simulink model "solargrid"  (R2021a)
settings: Solver=ode4  StartTime=0.0  StopTime=2.5  RelTol=1e-3
PreLoadFcn:
  | Ts_Power=1e-6;
  | Ts_Control=100e-6;
InitFcn:
  | Ts_Power=1e-6;
  | Ts_Control=100e-6;
undefined symbols (not defined in the file): D1, Delta, sigbuilder_block
libraries: spsSeriesRLCBranchLib x5, spsVoltageMeasurementLib x3, spsThreePhaseTransformerTwoWindingsLib x2, spsDistributedParametersLineLib x2, spsThreePhaseParallelRLCLoadLib x2, pid_lib x2, spsabctodq0Lib x2, spsThreePhaseSeriesRLCLoadLib x1, spsThreeLevelBridgeLib x1, spsThreePhaseSourceLib x1, spsGroundLib x1, spsGroundingTransformerLib x1
(part 1 of 2)
settings Model: SimulationMode=accelerator  Creator=The MathWorks, Inc.  LastModifiedBy=aks
settings SolverCC: AlgebraicLoopSolver=TrustRegion
settings DataIOCC: LimitDataPoints=on  SaveFormat=Array  SignalLogging=off  DSMLogging=off  ReturnWorkspaceOutputs=off
settings OptimizationCC: ExpressionDepthLimit=2147483647  EfficientMapNaN2IntZero=off  LifeSpan=inf
settings DebuggingCC: UnderspecifiedInitializationDetection=Classic  MergeDetectMultiDrivingBlocksExec=none  SolverPrmCheckMsg=warning  FcnCallInpInsideContextMsg=warning  StateNameClashWarn=warning  SFUnexpectedBacktrackingDiag=warning  SFNoUnconditionalDefaultTransitionDiag=warning  SFExecutionAtInitializationDiag=none  SFMachineParentedDataDiag=warning  ArithmeticOperatorsInVariantConditions=warning
settings HardwareCC: ProdBitPerPointer=32  ProdBitPerSizeT=32  ProdBitPerPtrDiffT=32  ProdLargestAtomicFloat=None  ProdIntDivRoundTo=Undefined  ProdEndianess=Unspecified  ProdWordSize=32  ProdHWDeviceType=32-bit Generic  TargetBitPerLong=64  TargetBitPerPointer=64  TargetBitPerSizeT=64  TargetBitPerPtrDiffT=64  TargetLongLongMode=on  TargetIntDivRoundTo=Zero  TargetEndianess=LittleEndian  TargetWordSize=64  TargetHWDeviceType=MATLAB Host  ProdEqTarget=off
settings ModelReferenceCC: PropagateSignalLabelsOutOfModel=off
settings SFSimCC: SimUseLocalCustomCode=off  CustomCodeUndefinedFunction=UseInterfaceOnly
settings CodeAppCC: MaxIdLength=128
settings GRTTargetCC: TargetLangStandard=C89/C90 (ANSI)  CombineOutputUpdateFcns=off  GRTInterface=on
settings ConfigComp: CovMetricSettings=dw  CovSaveCumulativeToWorkspaceVar=on  CovSaveSingleToWorkspaceVar=on  CovExternalEMLEnable=off  CovSFcnEnable=off
settings SimscapeCC: SimscapeNormalizeSystem=off

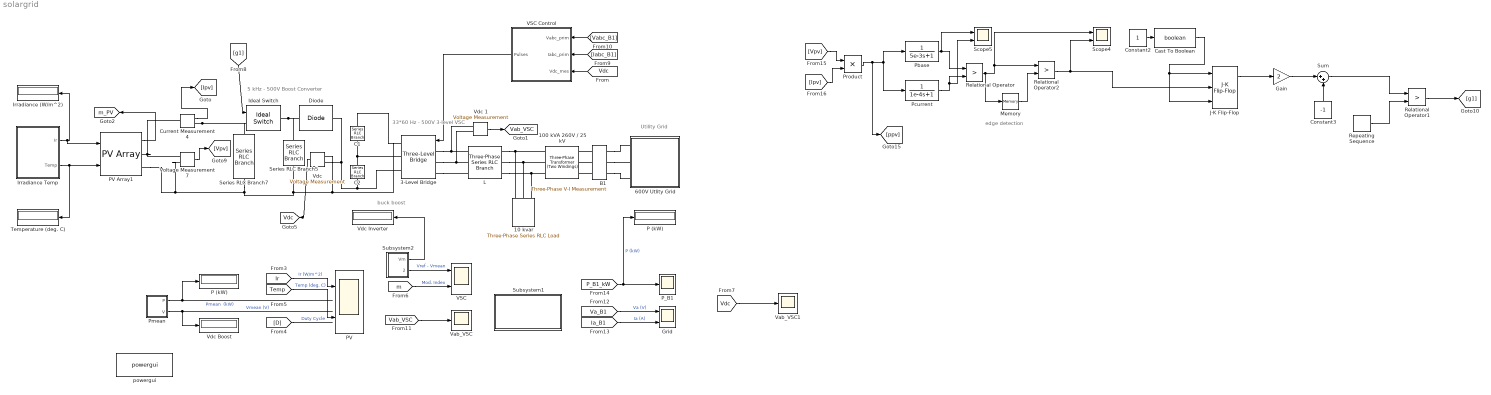
== system solargrid ==
  note: 5 kHz - 500V
      | Boost Converter
  note: 33*60 Hz - 500V
      | 3-level VSC
  note: Utility Grid
  note: buck boost
  note: edge detection
  10 kvar : spsThreePhaseSeriesRLCLoadLib/Three-Phase Series RLC Load  LConnTagsString=A|B|C  Configuration=Y (grounded)  NominalVoltage=240  Vabc=[1e3 1e3 1e3]  Vabcp=[1e3 1e3 1e3]  NominalFrequency=60  UnbalancedPower=off  ActivePower=10e3/100  InductivePower=0  CapacitivePower=10e3  Pabc=[10e3 9e3 11e3]  QLabc=[100 90 110]  QCabc=[100 90 110]  Pabcp=[10e3 9e3 11e3]  QLabcp=[100 90 110]  QCabcp=[100 90 110]  Measurements=None  LoadType=constant Z
  100 kVA 260V / 25 kV : spsThreePhaseTransformerTwoWindingsLib/Three-Phase Transformer (Two Windings)  Winding1Connection=Yg  Winding2Connection=Delta (D1)  CoreType=Three single-phase transformers  SetSaturation=off  Hysteresis=off  DataFile='hysteresis'  SetInitialFlux=off  Measurements=None  UNITS=pu  NominalPower=[100e3 , 60 ]  Winding1=[ 25e3 , 0.001 , 0.03 ]  Winding2=[ 260 , 0.001 , 0.03 ]  Rm=500  Lm=500  L0=0.5  Saturation=[ 0,0 ; 0.0024,1.2 ; 1.0,1.52 ]  InitialFluxes=[ 0.8 , -0.8 , 0.7 ]  BreakLoop=off  DiscreteSolver=Trapezoidal iterative  DataType=off  TransfoNumber=0
  3-Level Bridge : spsThreeLevelBridgeLib/Three-Level Bridge  Arms=3  SnubberResistance=1e6  SbubberCapacitance=inf  Device=IGBT / Diodes  Ron=0.2e-3  ForwardVoltages="[  0  0 ]"  Measurements=None
      settings: AttributesFormatString=\n  SourceProductBaseCode=PS
  600V Utlity Grid : Subsystem
  B1 : spsThreePhaseVIMeasurementLib/Three-Phase V-I Measurement  VoltageMeasurement=phase-to-ground  SetLabelV=on  LabelV=Vabc_B1  Vpu=off  VpuLL=off  CurrentMeasurement=yes  SetLabelI=on  LabelI=Iabc_B1  Ipu=off  Pbase=100e6  Vbase=500e3  OutputType=Magnitude  PhasorSimulation=off  PSBequivalent=0
  C1 : spsSeriesRLCBranchLib/Series RLC Branch  LConnTagsString=__new0  RConnTagsString=__new0  BranchType=C  Resistance=1.0  Inductance=1.0  SetiL0=off  InitialCurrent=0  Capacitance=12000e-06  Setx0=off  InitialVoltage=0  Measurements=None
  C2 : spsSeriesRLCBranchLib/Series RLC Branch  LConnTagsString=__new0  RConnTagsString=__new0  BranchType=C  Resistance=1.0  Inductance=1.0  SetiL0=off  InitialCurrent=0  Capacitance=12000e-06  Setx0=off  InitialVoltage=0  Measurements=None
  Cast To Boolean : DataTypeConversion  OutDataTypeStr=boolean
  Constant2 : Constant
  Constant3 : Constant  Value=-1
  Current Measurement4 : spsCurrentMeasurementLib/Current Measurement  PhasorSimulation=off  OutputType=Complex  PSBequivalent=0
  Diode : spsDiodeLib/Diode  Ron=1e-5  Lon=0  Vf=0.8  IC=0  UseSnubber=0  Rs=500  Cs=250e-9  Measurements=off
  Gain : Gain  Gain=2
  Grid : Scope  NumInputPorts=2
  Ideal Switch : spsIdealSwitchLib/Ideal Switch  Ron=0.001  Lon=0  IC=0  Rs=1e5  Cs=inf  Measurements=off
  Irradiance (W/m^2) : Display
      settings: Format=bank  Decimation=1000
  Irradiance Temp : Subsystem  Tag=STV Subsys  LoadFcn=sigbuilder_block('load');  StartFcn=sigbuilder_block('start');  StopFcn=sigbuilder_block('stop');  ClipboardFcn=sigbuilder_block('clipboard');  mask(Sigbuilder block){tuvar=[0:10]}
      mask help: Sigbuilder GUI
      mask init:
      | if ~strcmp(get_param(bdroot(gcbh),'SimulationStatus'),'stopped') tuvar = sigbuilder_block('maskInit'); end
      settings: CopyFcn=sigbuilder_block('copy');  DeleteFcn=sigbuilder_block('delete');  ModelCloseFcn=sigbuilder_block('modelClose');  PreSaveFcn=sigbuilder_block('preSave');  PauseFcn=sigbuilder_block('pause')  ContinueFcn=sigbuilder_block('continue')  NameChangeFcn=sigbuilder_block('namechange');  OpenFcn=sigbuilder_block('open',[54 0 1386 674.25 ]);  CloseFcn=sigbuilder_block('close');
      mask Display: plot(0, 0, 100, 100,[2, 2, 32, 32, 2], [68, 8, 8, 68, 68],[32, 2], [38, 38], [32, 19, 2],[53, 60, 44], [32, 17, 17, 2],[16, 16, 31, 31]);txt = getActiveGroup(gcbh);text(2, 100, txt,'verticalAlignment', 'top');
  J-K Flip-Flop : simulink_extras/Flip Flops/J-K Flip-Flop  initial_condition=1
  L : spsThreePhaseSeriesRLCBranchLib/Three-Phase Series RLC Branch  LConnTagsString=A|B|C  RConnTagsString=A|B|C  BranchType=RL  Resistance=500e-6*377/50/2  Inductance=500e-6/2  Capacitance=inf  Measurements=None
  Memory : Memory  InheritSampleTime=on
  P (kW) : Display
      settings: Format=bank  Decimation=2000
  "P (kW) " : Display
      settings: Format=bank  Decimation=2000
  PV : Scope  NumInputPorts=2
  PV Array1 : spsPVArrayLib/PV Array  Npar=40  Nser=10  PlotType=array @ 1000 W/m2 & specified temperatures  S_vec="[ 1000  500  100 ]"  Temp_C_vec=[ 45 25]  ModuleName=User-defined  PlotWhenSelected=off  Pm=213.15  Ncell=60  Voc=36.3  Isc=7.84  Vm=29  Im=7.35  beta_Voc_pc=-0.36099  alpha_Isc_pc=0.102  beta_Voc=-0.13104  alpha_Isc=0.0079968  IL=7.8654  I0=2.9273e-10  nI=0.98119  Rsh=313.0553  Rs=0.39381  RobustModel=off  RobustCellTemperature=313.3991  BAL=on  Tc=1e-6  Tfilter=5e-5
  P_B1 : Scope
  Pbase : TransferFcn  Denominator=[5e-3 1]
  Pcurrent : TransferFcn  Denominator=[1e-4 1]
  Pmean : Subsystem
  Product : Product
  Relational Operator : RelationalOperator  Operator=>  OutDataTypeStr=boolean  RndMeth=Simplest
  Relational Operator1 : RelationalOperator  Operator=>  OutDataTypeStr=boolean  RndMeth=Simplest
  Relational Operator2 : RelationalOperator  Operator=>  OutDataTypeStr=boolean  RndMeth=Simplest
  Repeating Sequence : simulink/Sources/Repeating Sequence  rep_seq_t=[0 1/40e3 1/20e3 3/40e3 1/10e3]  rep_seq_y=[0 1 0 -1 0]
  Scope4 : Scope  NumInputPorts=2
  Scope5 : Scope  NumInputPorts=2
  Series RLC Branch5 : spsSeriesRLCBranchLib/Series RLC Branch  LConnTagsString=__new0  RConnTagsString=__new0  BranchType=L  Resistance=1  Inductance=10e-3  SetiL0=off  InitialCurrent=0  Capacitance=1e-6  Setx0=off  InitialVoltage=0  Measurements=None
  Series RLC Branch7 : spsSeriesRLCBranchLib/Series RLC Branch  LConnTagsString=__new0  RConnTagsString=__new0  BranchType=C  Resistance=1  Inductance=1e-3  SetiL0=off  InitialCurrent=0  Capacitance=100e-6  Setx0=off  InitialVoltage=0  Measurements=None
  Subsystem1 : Subsystem
      mask Display: disp('Open this block\nto display additional \nscopes & measurements')
  Subsystem2 : Subsystem
  Sum : Sum  Inputs=|++
  Temperature (deg. C) : Display
      settings: Format=bank  Decimation=1000
  VSC : Scope  NumInputPorts=2
  VSC Control : Subsystem  mask(VSC Main Controller){nom=[ 100e3  60 ], Vnom=[ 25e3 260 ], Vnom_dc=500, RLxfo=[0.002  0.06 ], RLchoke=[2e-3  250e-6  ], K_VDCreg=[7  800], K_Ireg=[0.3 20], Ts=Ts_Control}
      mask prompts: nom "Nominal power and frequency [ Pnom(VA)  Fnom(Hz) ]:"; Vnom "Nominal primary and secondary voltages (Vrms LL) [ Vnom_prim   Vnom_sec ]:"; Vnom_dc "Nominal DC bus voltage (V):"; RLxfo "Total transformer leakage impedance (pu/Pnom) [ Rxfo  Lxf ]"; RLchoke "Choke impedance [ R(ohm) L(H) ]"; K_VDCreg "VDC regultator gains [ Kp  Ki ]:"; K_Ireg "Current regulator gains [ Kp  Ki ]:"; Ts "Sample time"
      mask init:
      | Pnom=nom(1);
      | Fnom=nom(2);
      | Vnom_prim=Vnom(1);
      | Vnom_sec=Vnom(2);
      | Zbase=Vnom_sec^2/Pnom;
      | Rtot_pu=RLxfo(1) + RLchoke(1)/Zbase;
      | Ltot_pu=RLxfo(2) + RLchoke(2)/(Zbase/(2*pi*Fnom));
      | Kp_VDCreg=K_VDCreg(1);
      | Ki_VDCreg=K_VDCreg(2);
      | Kp_Ireg=K_Ireg(1);
      | Ki_Ireg=K_Ireg(2);
      | Vdc_ref=Vnom_dc;
      | % Used to determine initial value of Boost Control (MPPT)
      | assignin('base','Vdc_ref_Inv',Vdc_ref);
  Vab_VSC : Scope
  Vab_VSC1 : Scope
  "Vdc " : spsVoltageMeasurementLib/Voltage Measurement  Tag=PoWeRsYsTeMmEaSuReMeNt  PhasorSimulation=off  OutputType=Magnitude  PSBequivalent=0
  Vdc 1 : spsVoltageMeasurementLib/Voltage Measurement  Tag=PoWeRsYsTeMmEaSuReMeNt  PhasorSimulation=off  OutputType=Magnitude  PSBequivalent=0
  Vdc Boost : Display
      settings: Format=bank  Decimation=2000
  Vdc Inverter : Display
      settings: Format=bank  Decimation=2000
  Voltage Measurement7 : spsVoltageMeasurementLib/Voltage Measurement  PhasorSimulation=off  OutputType=Complex  PSBequivalent=0
  powergui : spspowerguiLib/powergui  Priority=1  SimulationMode=Discrete  SampleTime=1e-06  frequency=60  Iterations=50  frequencyindice=0  Pbase=100e6  ErrMax=1e-4  UnitsV=kV  UnitsW=MW  buscounter=0  FunctionMessages=off  echomessages=off  EnableUseOfTLC=off  CurrentSourceSwitches=off  DisableSnubberDevices=off  DisableRonSwitches=off  DisableVfSwitches=off  DisplayEquations=off  AutomaticDiscreteSolvers=off  SolverType=Tustin/Backward Euler (TBE)  Interpol=off  ExternalGateDelay=off  methode=off  Ts=0  x0status=blocks  SPID=off  SwTol=0  HookPort=off  NonlinearTolerance=1e-8  nMaxIteration=10  ContinueOnMaxIteration=off  RestoreLinks=warning  ResistiveCurrentMeasurement=off  Frange=[0:2:500]  Ylog=off  Xlog=on  ShowGrid=off  save=off  variable=ZData  structure=0  ZoomFFT=on  StartTime=0.0  cycles=1  DisplayStyle=1  fundamental=60  FreqAxis=off  MaxFrequency=1000  frequencyindicesteady=1  RmsSteady=1  display=off
  tag scope: Vab_VSC=global, Vdc=global, m_PV=global
  wires:
  "Vdc "/1 -> [Vdc]
  [Vabc_B1] -> VSC Control/1(Vabc_prim)
  [Iabc_B1] -> VSC Control/2(Iabc_prim)
  [Vdc] -> VSC Control/3(Vdc_mes)
  VSC Control/1(Pulses) -> 3-Level Bridge/1
  Pmean/1(P) -> "P (kW) "/1  "Pmean  (kW)"
  [m] -> VSC/2  "Mod. Index"
  Vdc 1/1 -> [Vab_VSC]
  [Vab_VSC] -> Vab_VSC/1
  [Ia_B1] -> Grid/2  "Ia (A)"
  [Va_B1] -> Grid/1  "Va (V)"
  [P_B1_kW] -> P_B1/1, P (kW)/1  "P (kW)"
  Pmean/2(V) -> Vdc Boost/1  "Vmean (V)"
  Subsystem2/2(VrVm) -> VSC/1  "Vref - Vmean"
  Subsystem2/1(Vm) -> Vdc Inverter/1
  Irradiance Temp/1(Ir) -> PV Array1/1, Irradiance (W/m^2)/1
  Irradiance Temp/2(Temp) -> PV Array1/2, Temperature (deg. C)/1
  [D] -> ?  "Duty Cycle"
  [Temp] -> PV/2  "Temp (deg. C)"
  [Ir] -> PV/1  "Ir (W/m^2)"
  PV Array1/1 -> [m_PV]
  [Vdc] -> Vab_VSC1/1
  Voltage Measurement7/1 -> [Vpv]
  [g1] -> Ideal Switch/1
  Current Measurement4/1 -> [Ipv]
  Relational Operator1/1 -> [g1]
  Product/1 -> [ppv], Pcurrent/1, Pbase/1
  [Vpv] -> Product/1
  Constant2/1 -> Cast To Boolean/1
  Relational Operator2/1 -> Scope4/2, J-K Flip-Flop/2
  Constant3/1 -> Sum/2
  Relational Operator/1 -> Scope4/1, Relational Operator2/1, Memory/1
  Pbase/1 -> Scope5/1, Relational Operator/1
  Memory/1 -> Relational Operator2/2
  Cast To Boolean/1 -> J-K Flip-Flop/3, J-K Flip-Flop/1
  [Ipv] -> Product/2
  Sum/1 -> Relational Operator1/1
  Gain/1 -> Sum/1
  Pcurrent/1 -> Scope5/2, Relational Operator/2
  Repeating Sequence/1 -> Relational Operator1/2
  J-K Flip-Flop/1 -> Gain/1
  connections:
  3-Level Bridge/LConn1 -- L/LConn1 -- Vdc 1/LConn1
  3-Level Bridge/LConn2 -- L/LConn2 -- Vdc 1/LConn2
  3-Level Bridge/LConn3 -- L/LConn3
  L/RConn1 -- 100 kVA 260V / 25 kV/RConn1 -- 10 kvar/LConn1
  L/RConn2 -- 100 kVA 260V / 25 kV/RConn2 -- 10 kvar/LConn2
  L/RConn3 -- 100 kVA 260V / 25 kV/RConn3 -- 10 kvar/LConn3
  B1/LConn1 -- 100 kVA 260V / 25 kV/LConn1
  B1/LConn2 -- 100 kVA 260V / 25 kV/LConn2
  B1/LConn3 -- 100 kVA 260V / 25 kV/LConn3
  C2/LConn1 -- C1/RConn1 -- 3-Level Bridge/RConn2
  B1/RConn2 -- 600V Utlity Grid/LConn2
  B1/RConn1 -- 600V Utlity Grid/LConn1
  B1/RConn3 -- 600V Utlity Grid/LConn3
  Current Measurement4/RConn1 -- Series RLC Branch7/LConn1 -- Ideal Switch/LConn1
  Ideal Switch/RConn1 -- Series RLC Branch5/LConn1 -- Diode/RConn1
  Voltage Measurement7/LConn1 -- PV Array1/RConn1 -- Current Measurement4/LConn1
  Voltage Measurement7/LConn2 -- Series RLC Branch7/RConn1 -- "Vdc "/LConn1 -- 3-Level Bridge/RConn1 -- C1/LConn1 -- Series RLC Branch5/RConn1 -- PV Array1/RConn2
  Diode/LConn1 -- "Vdc "/LConn2 -- C2/RConn1 -- 3-Level Bridge/RConn3

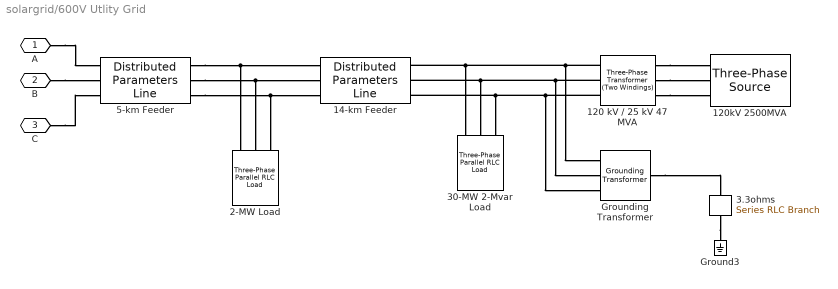
== system solargrid/600V Utlity Grid ==
  120 kV / 25 kV 47 MVA : spsThreePhaseTransformerTwoWindingsLib/Three-Phase Transformer (Two Windings)  Winding1Connection=Yg  Winding2Connection=Delta (D1)  CoreType=Three single-phase transformers  SetSaturation=off  Hysteresis=off  DataFile='basic_model'  SetInitialFlux=off  Measurements=None  UNITS=pu  NominalPower=[47e6 60 ]  Winding1="[ 120e3  0.08/30   0.08 ]"  Winding2="[ 25e3  0.08/30  0.08]"  Rm=500  Lm=500  L0=0.5  Saturation="[ 0,0  ;  0.005,1.2  ;  1.0,1.4 ]"  InitialFluxes=[ 0.8 , -0.8 , 0.7 ]  BreakLoop=off  DiscreteSolver=Trapezoidal iterative  DataType=off  TransfoNumber=0
  120kV 2500MVA : spsThreePhaseSourceLib/Three-Phase Source  InternalConnection=Yg  VoltagePhases=off  Voltage=120e3  PhaseAngle=0  Voltage_phases=[25e3 25e3 25e3]/sqrt(3)  PhaseAngles_phases=[0 -120 +120]  Frequency=60  NonIdealSource=on  SpecifyImpedance=on  Resistance=0.8929  Inductance=16.58e-3  ShortCircuitLevel=2500e6  BaseVoltage=120e3  XRratio=7  BusType=swing  Pref=0  Qref=0  Prefabc=[10e3, 10e3, 10e3]  Qrefabc=[0, 0, 0]  Qmin=-inf  Qmax=inf
  14-km Feeder : spsDistributedParametersLineLib/Distributed Parameters Line  Phases=3  Length=14  Frequency=60  Resistance=[0.1153 0.413]  Inductance=[1.05e-3 3.32e-3]  Capacitance=[11.33e-009 5.01e-009]  x1=[-5.8e-05 -4.281464951191e-09 0 0;-5.7e-05 -4.28163095328358e-09 0 0;-5.6e-05 -4.28179634686092e-09 0 0;-5.5e-05 -4.28196113189951e-09 0 0;-5.4e-05 -4.28212530837592e-09 0 0;-5.3e-05 -4.28228887626683e-09 0 0;-5.2e-05 -4.28245183554898e-09 0 0;-5.1e-05 -4.28261418619923e-09 0 0;-5e-05 -4.28277592819449e-09 0 0;-4.9e-05 -4.28293706151177e-09 -3790.73535189767 -24061.4134200266;-4.8e-05 -4.28309758612819e-09 -3781.66414358227 -24062.840783721;-4.7e-05 -4.28325750202091e-09 -3772.59239780806 -24064.2647275491;-4.6e-05 -4.28341680916722e-09 -3763.52011586434 -24065.6852513085;-4.5e-05 -4.28357550754448e-09 -3754.44729904048 -24067.1023547973;-4.4e-05 -4.28373359713012e-09 -3745.37394862592 -24068.5160378142;-4.3e-05 -4.28389107790169e-09 -3736.3000659102 -24069.9263001581;-4.2e-05 -4.2840479498368e-09 -3727.22565218291 -24071.3331416287;-4.1e-05 -4.28420421291315e-09 -3718.15070873374 -24072.7365620261;-4e-05 -4.28435986710853e-09 -3709.07523685243 -24074.1365611507;-3.9e-05 -4.28451491240084e-09 -3699.9992378288 -24075.5331388036;-3.8e-05 -4.28466934876802e-09 -3690.92271295277 -24076.9262947863;-3.7e-05 -4.28482317618813e-09 -3681.84566351431 -24078.3160289009;-3.6e-05 -4.2849763946393e-09 -3672.76809080347 -24079.7023409497;-3.5e-05 -4.28512900409978e-09 -3663.68999611037 -24081.0852307359;-3.4e-05 -4.28528100454785e-09 -3654.61138072522 -24082.4646980627;-3.3e-05 -4.28543239596192e-09 -3645.53224593829 -24083.8407427343;-3.2e-05 -4.28558317832048e-09 -3636.45259303993 -24085.213364555;-3.1e-05 -4.28573335160209e-09 -3627.37242332055 -24086.5825633297;-3e-05 -4.28588291578542e-09 -3618.29173807065 -24087.9483388638;-2.9e-05 -4.2860318708492e-09 -3609.2105385808 -24089.3106909633;-2.8e-05 -4.28618021677226e-09 -3600.12882614165 -24090.6696194346;-2.7e-05 -4.28632795353353e-09 -3591.0466020439 -24092.0251240844;-2.6e-05 -4.286475081112e-09 -3581.96386757834 -24093.3772047201;-2.5e-05 -4.28662159948677e-09 -3572.88062403583 -24094.7258611496;-2.4e-05 -4.28676750863701e-09 -3563.7968727073 -24096.0710931813;-2.3e-05 -4.28691280854198e-09 -3554.71261488376 -24097.4129006238;-2.2e-05 -4.28705749918104e-09 -3545.62785185628 -24098.7512832866;-2.1e-05 -4.28720158053362e-09 -3536.54258491601 -24100.0862409793;-2e-05 -4.28734505257924e-09 -3527.45681535417 -24101.4177735123;-1.9e-05 -4.28748791529752e-09 -3518.37054446204 -24102.7458806964;-1.8e-05 -4.28763016866814e-09 -3509.283773531 -24104.0705623427;-1.7e-05 -4.2877718126709e-09 -3500.19650385247 -24105.3918182631;-1.6e-05 -4.28791284728566e-09 -3491.10873671795 -24106.7096482696;-1.5e-05 -4.28805327249237e-09 -3482.02047341903 -24108.0240521751;-1.4e-05 -4.28819308827108e-09 -3472.93171524734 -24109.3350297928;-1.3e-05 -4.28833229460192e-09 -3463.8424634946 -24110.6425809363;-1.2e-05 -4.28847089146511e-09 -3454.7527194526 -24111.9467054197;-1.1e-05 -4.28860887884094e-09 -3445.66248441319 -24113.2474030578;-1e-05 -4.28874625670981e-09 -3436.5717596683 -24114.5446736656;-9e-06 -4.28888302505218e-09 -3427.48054650992 -24115.8385170589;-8e-06 -4.28901918384863e-09 -3418.38884623011 -24117.1289330537;-7e-06 -4.2891547330798e-09 -3409.29666012101 -24118.4159214666;-6e-06 -4.28928967272643e-09 -3400.20398947483 -24119.6994821147;-5e-06 -4.28942400276934e-09 -3391.11083558383 -24120.9796148156;-4e-06 -4.28955772318944e-09 -3382.01719974035 -24122.2563193874;-3e-06 -4.28969083396771e-09 -3372.9230832368 -24123.5295956486;-2e-06 -4.28982333508526e-09 -3363.82848736566 -24124.7994434182;-1e-06 -4.28995522652324e-09 -3354.73341341947 -24126.0658625158]  x2=[-5.8e-05 -4.62050791098548e-09 0 0;-5.7e-05 -4.62061598144239e-09 0 0;-5.6e-05 -4.62072339520672e-09 0 0;-5.5e-05 -4.6208301522632e-09 0 0;-5.4e-05 -4.62093625259667e-09 0 0;-5.3e-05 -4.62104169619204e-09 0 0;-5.2e-05 -4.62114648303433e-09 0 0;-5.1e-05 -4.62125061310864e-09 0 0;-5e-05 -4.62135408640018e-09 0 0;-4.9e-05 -4.62145690289425e-09 -3379.39242591114 -24244.0512732168;-4.8e-05 -4.62155906257621e-09 -3370.25239397934 -24245.3235513067;-4.7e-05 -4.62166056543157e-09 -3361.11188305951 -24246.5923835954;-4.6e-05 -4.62176141144589e-09 -3351.97089445072 -24247.8577699026;-4.5e-05 -4.62186160060484e-09 -3342.82942945211 -24249.1197100484;-4.4e-05 -4.62196113289418e-09 -3333.68748936289 -24250.3782038535;-4.3e-05 -4.62206000829977e-09 -3324.54507548233 -24251.6332511391;-4.2e-05 -4.62215822680755e-09 -3315.40218910977 -24252.8848517267;-4.1e-05 -4.62225578840356e-09 -3306.25883154462 -24254.1330054385;-4e-05 -4.62235269307394e-09 -3297.11500408636 -24255.3777120971;-3.9e-05 -4.62244894080492e-09 -3287.97070803452 -24256.6189715256;-3.8e-05 -4.62254453158282e-09 -3278.82594468872 -24257.8567835476;-3.7e-05 -4.62263946539405e-09 -3269.68071534863 -24259.0911479871;-3.6e-05 -4.62273374222511e-09 -3260.53502131399 -24260.3220646688;-3.5e-05 -4.62282736206262e-09 -3251.38886388461 -24261.5495334176;-3.4e-05 -4.62292032489326e-09 -3242.24224436036 -24262.7735540592;-3.3e-05 -4.62301263070382e-09 -3233.09516404117 -24263.9941264196;-3.2e-05 -4.62310427948119e-09 -3223.94762422707 -24265.2112503252;-3.1e-05 -4.62319527121234e-09 -3214.7996262181 -24266.4249256032;-3e-05 -4.62328560588433e-09 -3205.65117131441 -24267.6351520811;-2.9e-05 -4.62337528348434e-09 -3196.5022608162 -24268.8419295867;-2.8e-05 -4.6234643039996e-09 -3187.35289602373 -24270.0452579487;-2.7e-05 -4.62355266741748e-09 -3178.20307823734 -24271.245136996;-2.6e-05 -4.62364037372541e-09 -3169.0528087574 -24272.4415665581;-2.5e-05 -4.62372742291093e-09 -3159.90208888438 -24273.6345464649;-2.4e-05 -4.62381381496166e-09 -3150.75091991881 -24274.8240765469;-2.3e-05 -4.62389954986533e-09 -3141.59930316127 -24276.010156635;-2.2e-05 -4.62398462760976e-09 -3132.4472399124 -24277.1927865607;-2.1e-05 -4.62406904818285e-09 -3123.29473147291 -24278.3719661559;-2e-05 -4.6241528115726e-09 -3114.1417791436 -24279.547695253;-1.9e-05 -4.62423591776711e-09 -3104.98838422528 -24280.7199736848;-1.8e-05 -4.62431836675457e-09 -3095.83454801887 -24281.8888012849;-1.7e-05 -4.62440015852325e-09 -3086.68027182533 -24283.054177887;-1.6e-05 -4.62448129306155e-09 -3077.52555694568 -24284.2161033256;-1.5e-05 -4.62456177035791e-09 -3068.37040468102 -24285.3745774355;-1.4e-05 -4.62464159040092e-09 -3059.21481633249 -24286.529600052;-1.3e-05 -4.62472075317922e-09 -3050.05879320131 -24287.6811710111;-1.2e-05 -4.62479925868155e-09 -3040.90233658876 -24288.829290149;-1.1e-05 -4.62487710689678e-09 -3031.74544779616 -24289.9739573026;-1e-05 -4.62495429781382e-09 -3022.58812812493 -24291.1151723092;-9e-06 -4.62503083142172e-09 -3013.43037887651 -24292.2529350066;-8e-06 -4.62510670770958e-09 -3004.27220135243 -24293.3872452331;-7e-06 -4.62518192666664e-09 -2995.11359685428 -24294.5181028274;-6e-06 -4.62525648828219e-09 -2985.95456668368 -24295.645507629;-5e-06 -4.62533039254565e-09 -2976.79511214235 -24296.7694594775;-4e-06 -4.62540363944651e-09 -2967.63523453204 -24297.8899582131;-3e-06 -4.62547622897435e-09 -2958.47493515459 -24299.0070036768;-2e-06 -4.62554816111886e-09 -2949.31421531186 -24300.1205957096;-1e-06 -4.62561943586983e-09 -2940.15307630582 -24301.2307341534]  x3=[-5.8e-05 -1.8600557383193e-11 0 0;-5.7e-05 -1.86061131377125e-11 0 0;-5.6e-05 -1.86116662478883e-11 0 0;-5.5e-05 -1.86172167129313e-11 0 0;-5.4e-05 -1.86227645320527e-11 0 0;-5.3e-05 -1.86283097044638e-11 0 0;-5.2e-05 -1.86338522293767e-11 0 0;-5.1e-05 -1.86393921060037e-11 0 0;-5e-05 -1.86449293335573e-11 0 0;-4.9e-05 -1.86504639112507e-11 -23.5442847382522 -155.681477773836;-4.8e-05 -1.86559958382971e-11 -23.4855925321335 -155.690342696957;-4.7e-05 -1.86615251139106e-11 -23.4268969881884 -155.699185493008;-4.6e-05 -1.86670517373051e-11 -23.3681981147587 -155.708006160732;-4.5e-05 -1.86725757076953e-11 -23.3094959201869 -155.716804698877;-4.4e-05 -1.8678097024296e-11 -23.2507904128159 -155.72558110619;-4.3e-05 -1.86836156863226e-11 -23.1920816009891 -155.734335381426;-4.2e-05 -1.86891316929907e-11 -23.1333694930502 -155.743067523339;-4.1e-05 -1.86946450435164e-11 -23.0746540973437 -155.751777530689;-4e-05 -1.87001557371162e-11 -23.0159354222141 -155.760465402238;-3.9e-05 -1.87056637730067e-11 -22.9572134760069 -155.769131136751;-3.8e-05 -1.87111691504053e-11 -22.8984882670676 -155.777774732997;-3.7e-05 -1.87166718685294e-11 -22.8397598037425 -155.786396189746;-3.6e-05 -1.87221719265971e-11 -22.7810280943782 -155.794995505775;-3.5e-05 -1.87276693238266e-11 -22.7222931473217 -155.80357267986;-3.4e-05 -1.87331640594366e-11 -22.6635549709206 -155.812127710783;-3.3e-05 -1.87386561326462e-11 -22.6048135735229 -155.820660597328;-3.2e-05 -1.87441455426749e-11 -22.546068963477 -155.829171338281;-3.1e-05 -1.87496322887424e-11 -22.487321149132 -155.837659932435;-3e-05 -1.87551163700691e-11 -22.4285701388371 -155.846126378581;-2.9e-05 -1.87605977858755e-11 -22.3698159409422 -155.854570675517;-2.8e-05 -1.87660765353825e-11 -22.3110585637976 -155.862992822043;-2.7e-05 -1.87715526178115e-11 -22.2522980157539 -155.871392816961;-2.6e-05 -1.87770260323843e-11 -22.1935343051625 -155.879770659078;-2.5e-05 -1.87824967783229e-11 -22.1347674403749 -155.888126347204;-2.4e-05 -1.87879648548499e-11 -22.0759974297432 -155.89645988015;-2.3e-05 -1.8793430261188e-11 -22.0172242816199 -155.904771256733;-2.2e-05 -1.87988929965606e-11 -21.958448004358 -155.91306047577;-2.1e-05 -1.88043530601912e-11 -21.899668606311 -155.921327536085;-2e-05 -1.88098104513039e-11 -21.8408860958326 -155.929572436502;-1.9e-05 -1.8815265169123e-11 -21.7821004812773 -155.937795175848;-1.8e-05 -1.88207172128734e-11 -21.7233117709996 -155.945995752957;-1.7e-05 -1.88261665817801e-11 -21.664519973355 -155.954174166662;-1.6e-05 -1.88316132750686e-11 -21.6057250966988 -155.9623304158;-1.5e-05 -1.8837057291965e-11 -21.5469271493873 -155.970464499213;-1.4e-05 -1.88424986316954e-11 -21.4881261397769 -155.978576415745;-1.3e-05 -1.88479372934865e-11 -21.4293220762246 -155.986666164242;-1.2e-05 -1.88533732765654e-11 -21.3705149670877 -155.994733743556;-1.1e-05 -1.88588065801595e-11 -21.311704820724 -156.002779152538;-1e-05 -1.88642372034965e-11 -21.2528916454918 -156.010802390047;-9e-06 -1.88696651458048e-11 -21.1940754497497 -156.018803454941;-8e-06 -1.88750904063129e-11 -21.1352562418568 -156.026782346084;-7e-06 -1.88805129842496e-11 -21.0764340301726 -156.034739062342;-6e-06 -1.88859328788444e-11 -21.0176088230572 -156.042673602583;-5e-06 -1.88913500893269e-11 -20.9587806288708 -156.05058596568;-4e-06 -1.88967646149273e-11 -20.8999494559742 -156.058476150509;-3e-06 -1.8902176454876e-11 -20.8411153127287 -156.066344155948;-2e-06 -1.89075856084039e-11 -20.782278207496 -156.074189980879;-1e-06 -1.89129920747421e-11 -20.723438148638 -156.082013624187]  x4=[-5.8e-05 7.79859018799454e-12 0 0;-5.7e-05 7.80427695538787e-12 0 0;-5.6e-05 7.80996261361939e-12 0 0;-5.5e-05 7.81564716188105e-12 0 0;-5.4e-05 7.82133059936495e-12 0 0;-5.3e-05 7.82701292526334e-12 0 0;-5.2e-05 7.83269413876864e-12 0 0;-5.1e-05 7.83837423907342e-12 0 0;-5e-05 7.84405322537041e-12 0 0;-4.9e-05 7.8497310968525e-12 -1.3558136600917 -2.15298522697949;-4.8e-05 7.85540785271274e-12 -1.35500190745656 -2.15349620368187;-4.7e-05 7.86108349214434e-12 -1.35418996224543 -2.15400687432443;-4.6e-05 7.86675801434066e-12 -1.35337782457371 -2.15451723883456;-4.5e-05 7.87243141849522e-12 -1.35256549455682 -2.15502729713975;-4.4e-05 7.87810370380171e-12 -1.3517529723102 -2.1555370491675;-4.3e-05 7.88377486945396e-12 -1.35094025794934 -2.15604649484536;-4.2e-05 7.88944491464599e-12 -1.35012735158974 -2.15655563410093;-4.1e-05 7.89511383857194e-12 -1.34931425334694 -2.15706446686185;-4e-05 7.90078164042615e-12 -1.34850096333649 -2.1575729930558;-3.9e-05 7.90644831940308e-12 -1.34768748167397 -2.15808121261052;-3.8e-05 7.91211387469738e-12 -1.34687380847501 -2.15858912545376;-3.7e-05 7.91777830550384e-12 -1.34605994385525 -2.15909673151335;-3.6e-05 7.92344161101743e-12 -1.34524588793034 -2.15960403071714;-3.5e-05 7.92910379043326e-12 -1.344431640816 -2.16011102299304;-3.4e-05 7.9347648429466e-12 -1.34361720262793 -2.16061770826899;-3.3e-05 7.94042476775291e-12 -1.3428025734819 -2.16112408647297;-3.2e-05 7.94608356404777e-12 -1.34198775349367 -2.16163015753303;-3.1e-05 7.95174123102694e-12 -1.34117274277906 -2.16213592137723;-3e-05 7.95739776788635e-12 -1.34035754145389 -2.1626413779337;-2.9e-05 7.96305317382207e-12 -1.33954214963402 -2.16314652713059;-2.8e-05 7.96870744803035e-12 -1.33872656743533 -2.16365136889613;-2.7e-05 7.97436058970758e-12 -1.33791079497375 -2.16415590315855;-2.6e-05 7.98001259805033e-12 -1.3370948323652 -2.16466012984615;-2.5e-05 7.98566347225532e-12 -1.33627867972566 -2.16516404888728;-2.4e-05 7.99131321151944e-12 -1.33546233717111 -2.1656676602103;-2.3e-05 7.99696181503973e-12 -1.33464580481759 -2.16617096374365;-2.2e-05 8.0026092820134e-12 -1.33382908278113 -2.1666739594158;-2.1e-05 8.00825561163782e-12 -1.33301217117781 -2.16717664715526;-2e-05 8.01390080311053e-12 -1.33219507012374 -2.16767902689059;-1.9e-05 8.0195448556292e-12 -1.33137777973503 -2.16818109855038;-1.8e-05 8.0251877683917e-12 -1.33056030012785 -2.16868286206329;-1.7e-05 8.03082954059604e-12 -1.32974263141838 -2.16918431735799;-1.6e-05 8.03647017144041e-12 -1.32892477372282 -2.16968546436323;-1.5e-05 8.04210966012314e-12 -1.32810672715742 -2.17018630300777;-1.4e-05 8.04774800584273e-12 -1.32728849183843 -2.17068683322045;-1.3e-05 8.05338520779785e-12 -1.32647006788215 -2.17118705493011;-1.2e-05 8.05902126518733e-12 -1.32565145540488 -2.17168696806567;-1.1e-05 8.06465617721015e-12 -1.32483265452299 -2.17218657255608;-1e-05 8.07028994306548e-12 -1.32401366535282 -2.17268586833034;-9e-06 8.07592256195263e-12 -1.32319448801078 -2.17318485531748;-8e-06 8.08155403307107e-12 -1.3223751226133 -2.17368353344659;-7e-06 8.08718435562046e-12 -1.32155556927683 -2.17418190264678;-6e-06 8.09281352880059e-12 -1.32073582811783 -2.17467996284725;-5e-06 8.09844155181143e-12 -1.31991589925282 -2.17517771397719;-4e-06 8.10406842385312e-12 -1.31909578279832 -2.17567515596587;-3e-06 8.10969414412595e-12 -1.31827547887089 -2.17617228874258;-2e-06 8.11531871183038e-12 -1.31745498758712 -2.17666911223668;-1e-06 8.12094212616704e-12 -1.31663430906361 -2.17716562637756]  x5=5.70973484498186e-05  V1=[0 0 0 2.868e-09 2.436e+04 2.436e+04;0 0 0 377 377 377;1.571 1.571 1.571 -0.5389 -0.156 -1.727]  V2=[0 0 0 2.996e-09 2.448e+04 2.448e+04;0 0 0 377 377 377;1.571 1.571 1.571 -0.5232 -0.1382 -1.709]  I1=[0 0 0 1.022e-11 157.5 157.5;0 0 0 377 377 377;1.571 1.571 1.571 -1.198 -0.1498 -1.721]  I2=[0 0 0 6.231e-12 2.544 2.544;0 0 0 377 377 377;1.571 1.571 1.571 1.184 -0.5617 -2.133]  nHarmo=2  Measurements=None  Decoupling=off  VsMag0=0  VrMag0=0  VsAngle0=0  VrAngle0=0  IsMag0=0  IrMag0=0  IsAngle0=0  IrAngle0=0
      settings: SourceProductBaseCode=PS
  2-MW Load : spsThreePhaseParallelRLCLoadLib/Three-Phase Parallel RLC Load  LConnTagsString=A|B|C  Configuration=Y (grounded)  NominalVoltage=25e3  Vabc=[1e3 1e3 1e3]  Vabcp=[1e3 1e3 1e3]  NominalFrequency=60  UnbalancedPower=off  ActivePower=2e6  InductivePower=0  CapacitivePower=0  Pabc=[10e3 9e3 11e3]  QLabc=[100 90 110]  QCabc=[100 90 110]  Pabcp=[10e3 9e3 11e3]  QLabcp=[100 90 110]  QCabcp=[100 90 110]  Measurements=None  LoadType=constant Z
  "3.3ohms " : spsSeriesRLCBranchLib/Series RLC Branch  LConnTagsString=__new0  RConnTagsString=__new0  BranchType=R  Resistance=3.3  Inductance=[]  SetiL0=off  InitialCurrent=0  Capacitance=[]  Setx0=off  InitialVoltage=0  Measurements=None
  30-MW 2-Mvar Load : spsThreePhaseParallelRLCLoadLib/Three-Phase Parallel RLC Load  LConnTagsString=A|B|C  Configuration=Y (grounded)  NominalVoltage=25e3  Vabc=[1e3 1e3 1e3]  Vabcp=[1e3 1e3 1e3]  NominalFrequency=60  UnbalancedPower=off  ActivePower=30e6  InductivePower=2e6  CapacitivePower=0  Pabc=[10e3 9e3 11e3]  QLabc=[100 90 110]  QCabc=[100 90 110]  Pabcp=[10e3 9e3 11e3]  QLabcp=[100 90 110]  QCabcp=[100 90 110]  Measurements=None  LoadType=constant Z
  5-km Feeder : spsDistributedParametersLineLib/Distributed Parameters Line  Phases=3  Length=5  Frequency=60  Resistance=[0.1153 0.413]  Inductance=[1.05e-3 3.32e-3]  Capacitance=[11.33e-009 5.01e-009]  x1=[-2.1e-05 -4.20648949590592e-09 -3537.17773129426 -24101.4118174706;-2e-05 -4.20662176056209e-09 -3528.09146195673 -24102.7435893539;-1.9e-05 -4.2067534273635e-09 -3519.00469119872 -24104.0719356999;-1.8e-05 -4.20688449629143e-09 -3509.91742031166 -24105.3968563197;-1.7e-05 -4.20701496732725e-09 -3500.82965058706 -24106.718351025;-1.6e-05 -4.20714484045242e-09 -3491.7413833165 -24108.036419628;-1.5e-05 -4.20727411564848e-09 -3482.65261979161 -24109.3510619413;-1.4e-05 -4.20740279289706e-09 -3473.56336130412 -24110.6622777783;-1.3e-05 -4.20753087217987e-09 -3464.4736091458 -24111.9700669523;-1.2e-05 -4.20765835347871e-09 -3455.38336460853 -24113.2744292778;-1.1e-05 -4.20778523677546e-09 -3446.29262898421 -24114.5753645691;-1e-05 -4.20791152205208e-09 -3437.20140356486 -24115.8728726415;-9e-06 -4.20803720929064e-09 -3428.10968964253 -24117.1669533105;-8e-06 -4.20816229847326e-09 -3419.01748850936 -24118.4576063923;-7e-06 -4.20828678958217e-09 -3409.92480145755 -24119.7448317033;-6e-06 -4.20841068259968e-09 -3400.83162977939 -24121.0286290607;-5e-06 -4.20853397750817e-09 -3391.7379747672 -24122.308998282;-4e-06 -4.20865667429012e-09 -3382.64383771341 -24123.5859391852;-3e-06 -4.20877877292811e-09 -3373.54921991049 -24124.8594515888;-2e-06 -4.20890027340476e-09 -3364.45412265099 -24126.1295353119;-1e-06 -4.20902117570283e-09 -3355.35854722752 -24127.396190174]  x2=[-2.1e-05 -4.28629031427724e-09 -3536.54258491601 -24100.0862409793;-2e-05 -4.28643386938836e-09 -3527.45681535417 -24101.4177735123;-1.9e-05 -4.28657681530164e-09 -3518.37054446204 -24102.7458806964;-1.8e-05 -4.28671915199675e-09 -3509.283773531 -24104.0705623427;-1.7e-05 -4.28686087945348e-09 -3500.19650385247 -24105.3918182631;-1.6e-05 -4.28700199765166e-09 -3491.10873671795 -24106.7096482696;-1.5e-05 -4.28714250657126e-09 -3482.02047341903 -24108.0240521751;-1.4e-05 -4.28728240619229e-09 -3472.93171524734 -24109.3350297928;-1.3e-05 -4.28742169649489e-09 -3463.8424634946 -24110.6425809363;-1.2e-05 -4.28756037745924e-09 -3454.7527194526 -24111.9467054197;-1.1e-05 -4.28769844906564e-09 -3445.66248441319 -24113.2474030578;-1e-05 -4.28783591129447e-09 -3436.5717596683 -24114.5446736656;-9e-06 -4.28797276412619e-09 -3427.48054650992 -24115.8385170589;-8e-06 -4.28810900754135e-09 -3418.38884623011 -24117.1289330537;-7e-06 -4.28824464152059e-09 -3409.29666012101 -24118.4159214666;-6e-06 -4.28837966604463e-09 -3400.20398947483 -24119.6994821147;-5e-06 -4.28851408109428e-09 -3391.11083558383 -24120.9796148156;-4e-06 -4.28864788665044e-09 -3382.01719974035 -24122.2563193874;-3e-06 -4.2887810826941e-09 -3372.9230832368 -24123.5295956486;-2e-06 -4.28891366920631e-09 -3363.82848736566 -24124.7994434182;-1e-06 -4.28904564616824e-09 -3354.73341341947 -24126.0658625158]  x3=[-2.1e-05 -5.26881881757518e-12 -11.1569792961267 -79.1361755515072;-2e-05 -5.27407722779128e-12 -11.1271448686761 -79.140376010003;-1.9e-05 -5.27933488844339e-12 -11.09730885981 -79.1445652208864;-1.8e-05 -5.28459179878427e-12 -11.0674712737689 -79.1487431835621;-1.7e-05 -5.2898479580668e-12 -11.0376321147932 -79.1529098974362;-1.6e-05 -5.29510336554396e-12 -11.0077913871239 -79.1570653619165;-1.5e-05 -5.30035802046884e-12 -10.977949095002 -79.1612095764125;-1.4e-05 -5.30561192209465e-12 -10.9481052426686 -79.1653425403353;-1.3e-05 -5.31086506967467e-12 -10.9182598343654 -79.1694642530973;-1.2e-05 -5.31611746246233e-12 -10.8884128743339 -79.1735747141128;-1.1e-05 -5.32136909971113e-12 -10.8585643668161 -79.1776739227977;-1e-05 -5.32661998067471e-12 -10.8287143160542 -79.1817618785693;-9e-06 -5.3318701046068e-12 -10.7988627262904 -79.1858385808467;-8e-06 -5.33711947076124e-12 -10.7690096017674 -79.1899040290504;-7e-06 -5.34236807839198e-12 -10.739154946728 -79.1939582226027;-6e-06 -5.34761592675306e-12 -10.7092987654152 -79.1980011609273;-5e-06 -5.35286301509867e-12 -10.6794410620722 -79.2020328434498;-4e-06 -5.35810934268306e-12 -10.6495818409424 -79.206053269597;-3e-06 -5.36335490876061e-12 -10.6197211062696 -79.2100624387977;-2e-06 -5.36859971258583e-12 -10.5898588622975 -79.2140603504819;-1e-06 -5.37384375341329e-12 -10.5599951132704 -79.2180470040816]  x4=[-2.1e-05 -7.11060290285366e-12 -12.5606324025988 -78.900078757712;-2e-05 -7.10588252750641e-12 -12.5308868817952 -78.9048083977271;-1.9e-05 -7.10116114225478e-12 -12.5011395800731 -78.9095268236092;-1.8e-05 -7.09643874776978e-12 -12.4713905016603 -78.9142340346877;-1.7e-05 -7.09171534472258e-12 -12.4416396507848 -78.9189300302937;-1.6e-05 -7.08699093378447e-12 -12.4118870316748 -78.9236148097596;-1.5e-05 -7.0822655156269e-12 -12.3821326485589 -78.9282883724198;-1.4e-05 -7.07753909092145e-12 -12.3523765056657 -78.93295071761;-1.3e-05 -7.07281166033985e-12 -12.3226186072244 -78.9376018446675;-1.2e-05 -7.06808322455398e-12 -12.2928589574642 -78.9422417529314;-1.1e-05 -7.06335378423585e-12 -12.2630975606146 -78.9468704417421;-1e-05 -7.05862334005763e-12 -12.2333344209053 -78.951487910442;-9e-06 -7.05389189269161e-12 -12.2035695425663 -78.9560941583746;-8e-06 -7.04915944281024e-12 -12.173802929828 -78.9606891848854;-7e-06 -7.04442599108611e-12 -12.1440345869208 -78.9652729893213;-6e-06 -7.03969153819193e-12 -12.1142645180754 -78.9698455710309;-5e-06 -7.0349560848006e-12 -12.0844927275229 -78.9744069293643;-4e-06 -7.03021963158511e-12 -12.0547192194944 -78.9789570636731;-3e-06 -7.02548217921863e-12 -12.0249439982215 -78.9834959733108;-2e-06 -7.02074372837445e-12 -11.9951670679359 -78.9880236576323;-1e-06 -7.01600427972601e-12 -11.9653884328696 -78.992540115994]  x5=2.03919101606495e-05  V1=[0 0 0 2.827e-09 2.436e+04 2.436e+04;0 0 0 377 377 377;1.571 1.571 1.571 -0.5179 -0.1443 -1.715]  V2=[0 0 0 2.868e-09 2.436e+04 2.436e+04;0 0 0 377 377 377;1.571 1.571 1.571 -0.5251 -0.1443 -1.715]  I1=[0 0 0 7.018e-12 79.92 79.92;0 0 0 377 377 377;1.571 1.571 1.571 -1.622 -0.1386 -1.709]  I2=[0 0 0 7.946e-12 79.89 79.89;0 0 0 377 377 377;1.571 1.571 1.571 0.3547 -0.1565 -1.727]  nHarmo=2  Measurements=None  Decoupling=off  VsMag0=0  VrMag0=0  VsAngle0=0  VrAngle0=0  IsMag0=0  IrMag0=0  IsAngle0=0  IrAngle0=0
      settings: SourceProductBaseCode=PS
  Ground3 : spsGroundLib/Ground  LConnTagsString=a
  "Grounding Transformer " : spsGroundingTransformerLib/Grounding Transformer   UNITS=pu  NominalPower="[100e6   60]"  NominalVoltage=25e3  ZeroSequenceImpedance_pu=[0.025 0.75]  MagnetizationBranch_pu=[500 500]  ZeroSequenceImpedance_SI=[0.052083 589.05]  MagnetizationBranch_SI=[1041.7 3.927e+005]  Measurements=None
      settings: SourceProductBaseCode=PS
  A : PMIOPort  Side=Left
  B : PMIOPort  Port=2  Side=Left
  C : PMIOPort  Port=3  Side=Left
  connections:
  "3.3ohms "/RConn1 -- Ground3/LConn1
  120 kV / 25 kV 47 MVA/LConn1 -- 120kV 2500MVA/RConn1
  120 kV / 25 kV 47 MVA/LConn2 -- 120kV 2500MVA/RConn2
  120 kV / 25 kV 47 MVA/LConn3 -- 120kV 2500MVA/RConn3
  120 kV / 25 kV 47 MVA/RConn1 -- "Grounding Transformer "/LConn1 -- 14-km Feeder/RConn1 -- 30-MW 2-Mvar Load/LConn1
  120 kV / 25 kV 47 MVA/RConn2 -- "Grounding Transformer "/LConn2 -- 14-km Feeder/RConn2 -- 30-MW 2-Mvar Load/LConn2
  120 kV / 25 kV 47 MVA/RConn3 -- "Grounding Transformer "/LConn3 -- 14-km Feeder/RConn3 -- 30-MW 2-Mvar Load/LConn3
  5-km Feeder/RConn1 -- 14-km Feeder/LConn1 -- 2-MW Load/LConn1
  5-km Feeder/RConn2 -- 14-km Feeder/LConn2 -- 2-MW Load/LConn2
  5-km Feeder/RConn3 -- 14-km Feeder/LConn3 -- 2-MW Load/LConn3
  A/RConn1 -- 5-km Feeder/LConn1
  B/RConn1 -- 5-km Feeder/LConn2
  C/RConn1 -- 5-km Feeder/LConn3
  "Grounding Transformer "/RConn1 -- "3.3ohms "/LConn1

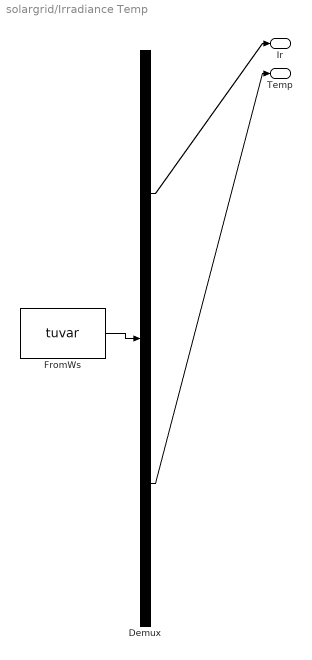
== system solargrid/Irradiance Temp ==
  Demux : Demux  Tag=STV Demux  Outputs=2
      settings: DisplayOption=none
  FromWs : FromWorkspace  Tag=STV FromWs  VariableName=tuvar
      SigBuilderData=|
      | common.afterFinalStr = 'Extrapolate'
      | common.sampleTime = '0'
      | dataSet(1).timeRange = [0 2]
      | dataSet(1).name = 'Constant Irradiance'
      | dataSet(2).timeRange = [0 2]
      | dataSet(2).name = 'Step Irradiance'
      | dataSet(3).timeRange = [0 3]
      | dataSet(3).name = 'Ramp-up/down Irradiance'
      | sbobj.Groups(1).Name = 'Constant Irradiance'
      | sbobj.Groups(1).Signals(1).Name = 'Ir'
      | sbobj.Groups(1).Signals(1).XData = [0 2]
      | sbobj.Groups(1).Signals(1).YData = [1000 1000]
      | sbobj.Groups(1).Signals(2).Name = 'Temp'
      | sbobj.Groups(1).Signals(2).XData = [0 1 1 2]
      | sbobj.Groups(1).Signals(2).YData = [0 0 1 1]
      | sbobj.Groups(1).TimeRange = [0 2]
      | sbobj.Groups(2).Name = 'Step Irradiance'
      | sbobj.Groups(2).Signals(1).Name = 'Ir'
      | sbobj.Groups(2).Signals(1).XData = [0 0.252 0.252 2]
      | sbobj.Groups(2).Signals(1).YData = [600 600 1000 1000]
      | sbobj.Groups(2).Signals(2).Name = 'Temp'
      | sbobj.Groups(2).Signals(2).XData = [0 1 1 2]
      | sbobj.Groups(2).Signals(2).YData = [0 0 1 1]
      | sbobj.Groups(2).TimeRange = [0 2]
      | sbobj.Groups(3).Name = 'Ramp-up/down Irradiance'
      | sbobj.Groups(3).Signals(1).Name = 'Ir'
      | sbobj.Groups(3).Signals(1).XData = [0 0.6 1.1 1.2 1.7 3]
      | sbobj.Groups(3).Signals(1).YData = [1000 1000 250 250 1000 1000]
      | sbobj.Groups(3).Signals(2).Name = 'Temp'
      | sbobj.Groups(3).Signals(2).XData = [0 2 2.1 3]
      | sbobj.Groups(3).Signals(2).YData = [25 25 50 50]
      | sbobj.Groups(3).TimeRange = [0 3]
  Ir : Outport  Tag=STV Outport  VectorParamsAs1DForOutWhenUnconnected=off
  Temp : Outport  Tag=STV Outport  Port=2  VectorParamsAs1DForOutWhenUnconnected=off
  wires:
  Demux/1 -> Ir/1
  FromWs/1 -> Demux/1
  Demux/2 -> Temp/1

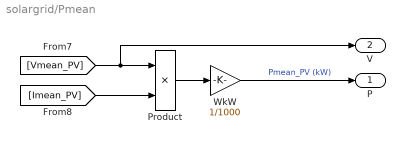
== system solargrid/Pmean ==
  Product : Product  RndMeth=Zero
  WkW : Gain  Gain=1/1000
  P : Outport  VectorParamsAs1DForOutWhenUnconnected=off
  V : Outport  Port=2  VectorParamsAs1DForOutWhenUnconnected=off
  wires:
  [Vmean_PV] -> Product/1, V/1
  Product/1 -> WkW/1
  [Imean_PV] -> Product/2
  WkW/1 -> P/1  "Pmean_PV (kW)"

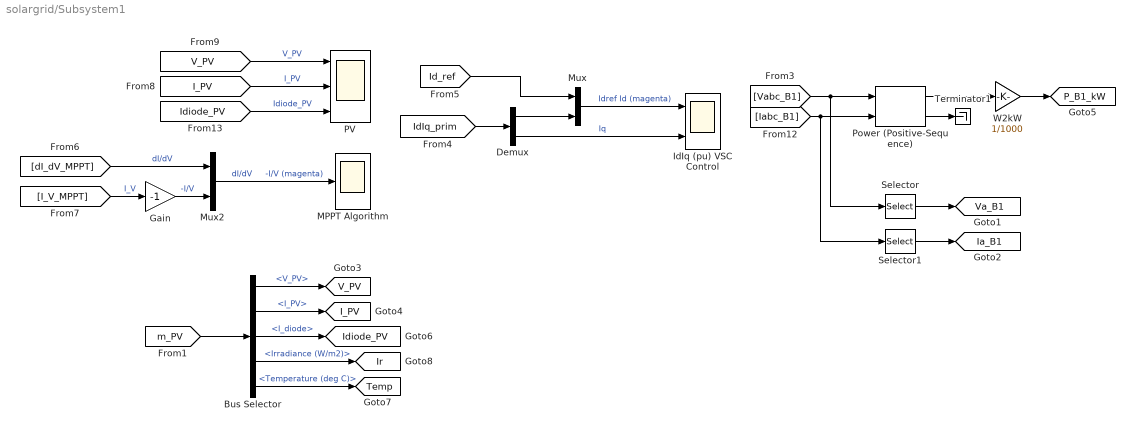
== system solargrid/Subsystem1 ==
  Bus Selector : BusSelector  OutputSignals=V_PV,I_PV,I_diode,Irradiance (W/m2),Temperature (deg C)
  Demux : Demux  Outputs=2
  Gain : Gain  Gain=-1
  IdIq (pu) VSC Control : Scope  NumInputPorts=2
  MPPT Algorithm : Scope
  Mux : Mux  Inputs=2
  Mux2 : Mux  Inputs=2
  PV : Scope  NumInputPorts=3
  Power (Positive-Sequence) : spsPowerPositiveSequenceLib/Power (Positive-Sequence)  Freq=60  Vinit=[0, 0]  Iinit=[0, 0]  Ts=Ts_Control
      settings: SourceProductBaseCode=PS
  Selector : Selector  InputPortWidth=3  IndexOptions=Index vector (dialog)  Indices=[1]  OutputSizes=1
  Selector1 : Selector  InputPortWidth=3  IndexOptions=Index vector (dialog)  Indices=[1]  OutputSizes=1
  Terminator1 : Terminator
  W2kW : Gain  Gain=1/1000
  tag scope: I_PV=global, Ia_B1=global, Idiode_PV=global, Ir=global, P_B1_kW=global, Temp=global, V_PV=global, Va_B1=global
  wires:
  [Vabc_B1] -> Power (Positive-Sequence)/1, Selector/1
  [Iabc_B1] -> Power (Positive-Sequence)/2, Selector1/1
  Power (Positive-Sequence)/1 -> W2kW/1
  [I_V_MPPT] -> Gain/1  "I_V"
  [IdIq_prim] -> Demux/1
  [Id_ref] -> Mux/1
  Demux/1 -> Mux/2
  Mux/1 -> IdIq (pu) VSC Control/1  "Idref Id (magenta)"
  Demux/2 -> IdIq (pu) VSC Control/2  "Iq"
  Selector/1 -> [Va_B1]
  Selector1/1 -> [Ia_B1]
  [V_PV] -> PV/1  "V_PV"
  [I_PV] -> PV/2  "I_PV"
  [Idiode_PV] -> PV/3  "Idiode_PV"
  [dI_dV_MPPT] -> Mux2/1  "dI/dV"
  Gain/1 -> Mux2/2  "-I/V"
  Mux2/1 -> MPPT Algorithm/1  "dI/dV     -I/V (magenta)"
  W2kW/1 -> [P_B1_kW]
  [m_PV] -> Bus Selector/1
  Bus Selector/1 -> [V_PV]  "<V_PV>"
  Bus Selector/2 -> [I_PV]  "<I_PV>"
  Bus Selector/4 -> [Ir]  "<Irradiance (W/m2)>"
  Bus Selector/3 -> [Idiode_PV]  "<I_diode>"
  Bus Selector/5 -> [Temp]  "<Temperature (deg C)>"
  Power (Positive-Sequence)/2 -> Terminator1/1

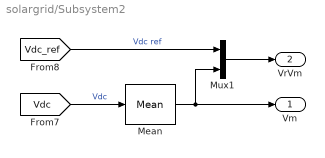
== system solargrid/Subsystem2 ==
  Mean : spsMeanLib/Mean  Freq=60  Vinit=0  Ts=Ts_Control
  Mux1 : Mux  Inputs=2
  Vm : Outport  VectorParamsAs1DForOutWhenUnconnected=off
  VrVm : Outport  Port=2  VectorParamsAs1DForOutWhenUnconnected=off
  wires:
  [Vdc_ref] -> Mux1/1  "Vdc ref"
  [Vdc] -> Mean/1  "Vdc"
  Mux1/1 -> VrVm/1
  Mean/1 -> Mux1/2, Vm/1

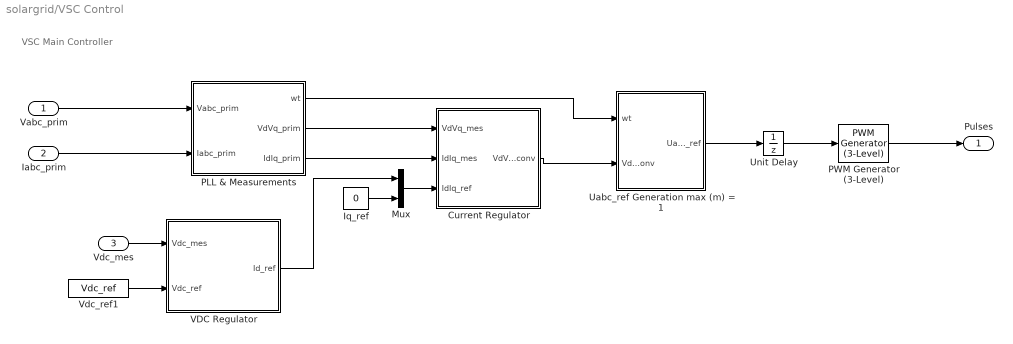
== system solargrid/VSC Control ==
  note: VSC Main Controller
  Vabc_prim : Inport  PortDimensions=3
  Iabc_prim : Inport  Port=2  PortDimensions=3
  Vdc_mes : Inport  Port=3  PortDimensions=1
  Current Regulator : Subsystem
  Iq_ref : Constant  Value=0
  Mux : Mux  Inputs=2
  PLL & Measurements : Subsystem
  PWM Generator (3-Level) : spsPWMGenerator3LevelLib/PWM Generator (3-Level)  ModulatorType=Three-phase bridge (12 pulses)  ModulatorMode=Unsynchronized  nF=27  Fc=33*60  ModulatingSignals=off  m=0.8  Freq=60  Phase=0  Ts=Ts_Power
      settings: SourceProductBaseCode=PS
  Uabc_ref Generation max (m) = 1 : Subsystem
  Unit Delay : UnitDelay  SampleTime=1e-4  HasFrameUpgradeWarning=on
  VDC Regulator : Subsystem
  Vdc_ref1 : Constant  Value=Vdc_ref
  Pulses : Outport  VectorParamsAs1DForOutWhenUnconnected=off
  wires:
  VDC Regulator/1(Id_ref) -> Mux/1
  PLL & Measurements/1(wt) -> Uabc_ref Generation max (m) = 1/1(wt)
  Current Regulator/1(VdVq_conv) -> Uabc_ref Generation max (m) = 1/2(VdVq_conv)
  Iq_ref/1 -> Mux/2
  Mux/1 -> Current Regulator/3(IdIq_ref)
  PLL & Measurements/3(IdIq_prim) -> Current Regulator/2(IdIq_mes)
  PLL & Measurements/2(VdVq_prim) -> Current Regulator/1(VdVq_mes)
  Vdc_mes/1 -> VDC Regulator/1(Vdc_mes)
  Vabc_prim/1 -> PLL & Measurements/1(Vabc_prim)
  Iabc_prim/1 -> PLL & Measurements/2(Iabc_prim)
  Unit Delay/1 -> PWM Generator (3-Level)/1
  PWM Generator (3-Level)/1 -> Pulses/1
  Uabc_ref Generation max (m) = 1/1(Uabc_ref) -> Unit Delay/1
  Vdc_ref1/1 -> VDC Regulator/2(Vdc_ref)

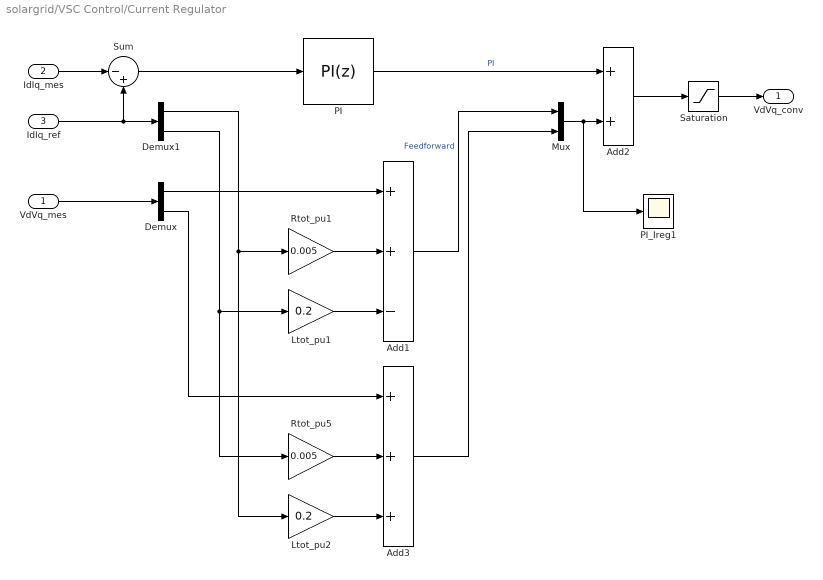
== system solargrid/VSC Control/Current Regulator ==
  VdVq_mes : Inport  PortDimensions=2
  IdIq_mes : Inport  Port=2  PortDimensions=2
  IdIq_ref : Inport  Port=3  PortDimensions=2
  Add1 : Sum  Inputs=++-
  Add2 : Sum
  Add3 : Sum  Inputs=+++
  Demux : Demux  Outputs=2
  Demux1 : Demux  Outputs=2
  Ltot_pu1 : Gain  Gain=0.2  SaturateOnIntegerOverflow=on  OutDataTypeStr=Inherit: Same as input  ParamDataTypeStr=Inherit: Same as input
  Ltot_pu2 : Gain  Gain=0.2  SaturateOnIntegerOverflow=on  OutDataTypeStr=Inherit: Same as input  ParamDataTypeStr=Inherit: Same as input
  Mux : Mux  Inputs=2
  PI : pid_lib/PID Controller  Controller=PI  Form=Parallel  TimeDomain=Discrete-time  UseExternalTs=off  SampleTime=Ts  IntegratorMethod=Forward Euler  FilterMethod=Forward Euler  ControllerParametersSource=internal  P=0.3  I=20  D=0  UseFilter=on  N=100  TunerSelectOption=Transfer Function Based (PID Tuner App)  InitialConditionSource=internal  InitialConditionForIntegrator=0  InitialConditionForFilter=0  DifferentiatorICPrevScaledInput=0  ExternalReset=none  TrackingMode=off  Kt=1  LimitOutput=on  SatLimitsSource=internal  UpperSaturationLimit=2  LowerSaturationLimit=-2  LinearizeAsGain=off  AntiWindupMode=none  Kb=1  POutMin=[]  POutMax=[]  IOutMin=[]  IOutMax=[]  DOutMin=[]  DOutMax=[]  NOutMin=[]  NOutMax=[]  SumOutMin=[]  SumOutMax=[]  SaturationOutMin=[]  SaturationOutMax=[]  PParamMin=[]  PParamMax=[]  IParamMin=[]  IParamMax=[]  DParamMin=[]  DParamMax=[]  NParamMin=[]  NParamMax=[]  KbParamMin=[]  KbParamMax=[]  KtParamMin=[]  KtParamMax=[]  KbOutMin=[]  KbOutMax=[]  KtOutMin=[]  KtOutMax=[]  IntegratorOutMin=[]  IntegratorOutMax=[]  FilterOutMin=[]  FilterOutMax=[]  SumI1OutMin=[]  SumI1OutMax=[]  SumI2OutMin=[]  SumI2OutMax=[]  SumI3OutMin=[]  SumI3OutMax=[]  SumI4OutMin=[]  SumI4OutMax=[]  SumDOutMin=[]  SumDOutMax=[]  DifferentiatorOutMin=[]  DifferentiatorOutMax=[]  FilterDiffOutCoefMin=[]  FilterDiffOutCoefMax=[]  ReciprocalOutMin=[]  ReciprocalOutMax=[]  SumDenOutMin=[]  SumDenOutMax=[]  SumNumOutMin=[]  SumNumOutMax=[]  DivideOutMin=[]  DivideOutMax=[]  UdiffTsProdOutMin=[]  UdiffTsProdOutMax=[]  NTsProdOutMin=[]  NTsProdOutMax=[]  UintegralTsProdOutMin=[]  UintegralTsProdOutMax=[]  UngainTsProdOutMin=[]  UngainTsProdOutMax=[]  IntegratorContinuousStateAttributes=''  IntegratorStateMustResolveToSignalObject=off  IntegratorRTWStateStorageClass=Auto  FilterContinuousStateAttributes=''  FilterStateMustResolveToSignalObject=off  FilterRTWStateStorageClass=Auto  ParallelPVariant=InternalParameters  IdealPVariant=Disabled  IVariant=InternalParameters  DVariant=Disabled  IntegratorVariant=Discrete  SatVariant=Enabled  AWVariant=Passthrough  PCopyVariant=Disabled  TRVariant=Disabled  FdbkBlocksVariant=Forward  IdealPFdbkVariant=Disabled  SatFdbkVariant=Disabled  DerivativeFilterVariant=Disabled  NVariant=Disabled  NCopyVariant=Disabled_SignalSpec  FilterICVariant=Disabled  IntegratorICVariant=InternalICs  ExternalResetVariant=Disabled  TRSumVariant=Passthrough  SumFdbkVariant=Disabled  SumVariant=Sum_PI  TsampFilterVariant=InternalTs  TsampNgainVariant=Passthrough  TsampIntegralVariant=Passthrough  ExternalSaturationOutDataTypeStr=Inherit: Same as second input
  PI_Ireg1 : Scope
  Rtot_pu1 : Gain  Gain=0.005  SaturateOnIntegerOverflow=on  OutDataTypeStr=Inherit: Same as input  ParamDataTypeStr=Inherit: Same as input
  Rtot_pu5 : Gain  Gain=0.005  SaturateOnIntegerOverflow=on  OutDataTypeStr=Inherit: Same as input  ParamDataTypeStr=Inherit: Same as input
  Saturation : Saturate  UpperLimit=2  LowerLimit=-2
  Sum : Sum  Inputs=|-+
  VdVq_conv : Outport  VectorParamsAs1DForOutWhenUnconnected=off
  wires:
  Mux/1 -> PI_Ireg1/1, Add2/2
  PI/1 -> Add2/1  "PI"
  Sum/1 -> PI/1
  IdIq_ref/1 -> Sum/2, Demux1/1
  IdIq_mes/1 -> Sum/1
  Add2/1 -> Saturation/1
  Saturation/1 -> VdVq_conv/1
  VdVq_mes/1 -> Demux/1
  Demux/1 -> Add1/1
  Rtot_pu1/1 -> Add1/2
  Demux1/1 -> Rtot_pu1/1, Ltot_pu2/1
  Ltot_pu1/1 -> Add1/3
  Demux1/2 -> Ltot_pu1/1, Rtot_pu5/1
  Rtot_pu5/1 -> Add3/2
  Ltot_pu2/1 -> Add3/3
  Add1/1 -> Mux/1  "Feedforward"
  Demux/2 -> Add3/1
  Add3/1 -> Mux/2

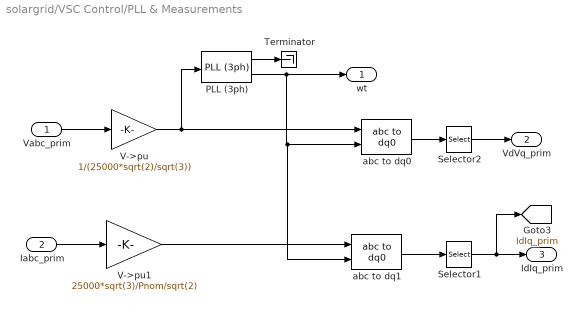
== system solargrid/VSC Control/PLL & Measurements ==
  Vabc_prim : Inport
  Iabc_prim : Inport  Port=2
  PLL (3ph) : spsPLL3phLib/PLL (3ph)  Fmin=45  Par_Init="[-0.57  Fnom]"  ParK=[180, 3200, 1]  TcD=1e-4  MaxRateChangeFreq=12  FilterCutOffFreq=25  Ts=Ts  AGC=on
  Selector1 : Selector  InputPortWidth=3  IndexOptions=Index vector (dialog)  Indices=[1 2]  OutputSizes=1
  Selector2 : Selector  InputPortWidth=3  IndexOptions=Index vector (dialog)  Indices=[1 2]  OutputSizes=1
  Terminator : Terminator
  V->pu : Gain  Gain=1/(25000*sqrt(2)/sqrt(3))  SaturateOnIntegerOverflow=on  OutDataTypeStr=Inherit: Same as input  ParamDataTypeStr=Inherit: Same as input
  V->pu1 : Gain  Gain=25000*sqrt(3)/Pnom/sqrt(2)  SaturateOnIntegerOverflow=on  OutDataTypeStr=Inherit: Same as input  ParamDataTypeStr=Inherit: Same as input
  abc to dq0 : spsabctodq0Lib/abc to dq0  Alignment=90 degrees behind phase A axis
  abc to dq1 : spsabctodq0Lib/abc to dq0  Alignment=90 degrees behind phase A axis
  wt : Outport  VectorParamsAs1DForOutWhenUnconnected=off
  VdVq_prim : Outport  Port=2  VectorParamsAs1DForOutWhenUnconnected=off
  IdIq_prim : Outport  Port=3  VectorParamsAs1DForOutWhenUnconnected=off
  tag scope: IdIq_prim=global
  wires:
  V->pu1/1 -> abc to dq1/1
  V->pu/1 -> PLL (3ph)/1, abc to dq0/1
  abc to dq1/1 -> Selector1/1
  Vabc_prim/1 -> V->pu/1
  Iabc_prim/1 -> V->pu1/1
  abc to dq0/1 -> Selector2/1
  Selector2/1 -> VdVq_prim/1
  Selector1/1 -> [IdIq_prim], IdIq_prim/1
  PLL (3ph)/2 -> wt/1, abc to dq1/2, abc to dq0/2
  PLL (3ph)/1 -> Terminator/1
